simulink model "dc_motor"  (R2022b)
settings: Solver=VariableStepAuto  StartTime=0.0  StopTime=10.0  MaxStep=15e-3  RelTol=1e-3
model workspace (MAT data in the model file):
  J = 7.1e-06
  L_a = 0.0089
  R_a = 5.95
  T_0 = 0.001
  b = 0.001
  k_e = 0.0514
  k_p = 2
  k_t = 0.0514
libraries: simulink x1
settings Model: Creator=Oleg  LastModifiedBy=Oleg
settings DataIOCC: ReturnWorkspaceOutputsName=SDOSimTest_Log
settings DebuggingCC: UnconnectedInputMsg=warning  UnconnectedOutputMsg=warning  UnconnectedLineMsg=warning
settings ModelReferenceCC: EnableRefExpFcnMdlSchedulingChecks=on
settings RTWCC: DLArmComputeVersion=19.05

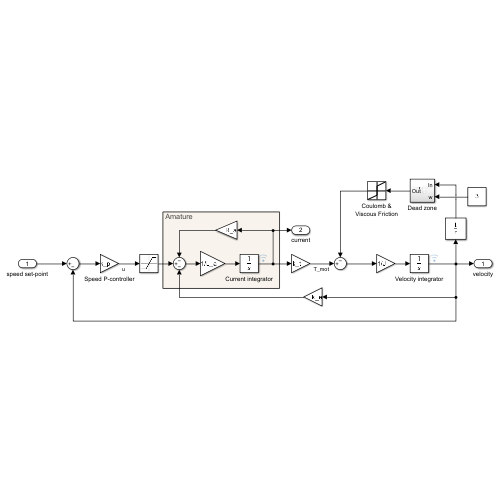
[thumbnail: Simulink's stored preview of the top-level diagram]
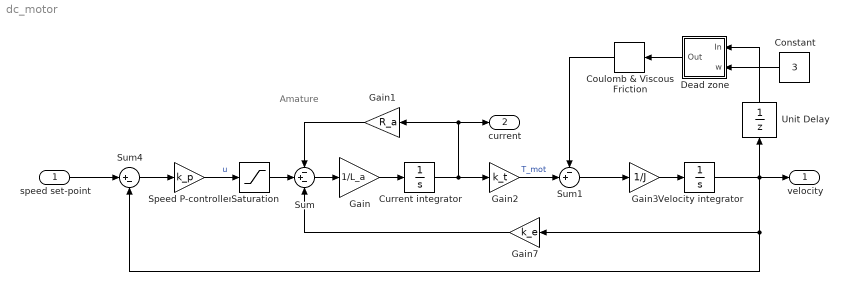
== system dc_motor ==
  note: Amature
  speed set-point : Inport
  Constant : Constant  Value=3
  Coulomb & Viscous Friction : simulink/Discontinuities/Coulomb & Viscous Friction  offset=T_0  gain=b
  Current integrator : Integrator
  Dead zone : Subsystem
  Gain : Gain  Gain=1/L_a
  Gain1 : Gain  Gain=R_a
  Gain2 : Gain  Gain=k_t
  Gain3 : Gain  Gain=1/J
  Gain7 : Gain  Gain=k_e
  Saturation : Saturate  UpperLimit=24  LowerLimit=-24
  Speed P-controller : Gain  Gain=k_p
  Sum : Sum  Inputs=-+-
  Sum1 : Sum  Inputs=-+|
  Sum4 : Sum  Inputs=|+-
  Unit Delay : UnitDelay  SampleTime=-1  HasFrameUpgradeWarning=on
  Velocity integrator : Integrator
  velocity : Outport
  current : Outport  Port=2
  wires:
  Gain/1 -> Current integrator/1
  Sum/1 -> Gain/1
  Gain1/1 -> Sum/1
  Current integrator/1 -> Gain2/1, current/1, Gain1/1
  Gain2/1 -> Sum1/2  "T_mot"
  Sum1/1 -> Gain3/1
  Gain3/1 -> Velocity integrator/1
  Velocity integrator/1 -> Unit Delay/1, velocity/1, Sum4/2, Gain7/1
  Gain7/1 -> Sum/3
  Sum4/1 -> Speed P-controller/1
  Constant/1 -> Dead zone/2(w)
  Unit Delay/1 -> Dead zone/1(In)
  Dead zone/1(Out) -> Coulomb & Viscous Friction/1
  Saturation/1 -> Sum/2
  Speed P-controller/1 -> Saturation/1  "u"
  speed set-point/1 -> Sum4/1
  Coulomb & Viscous Friction/1 -> Sum1/1

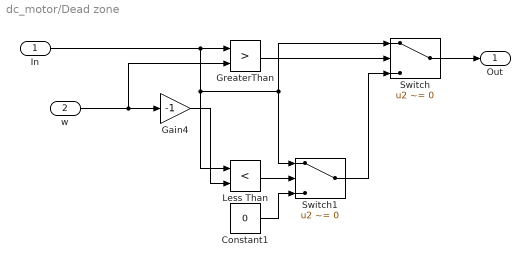
== system dc_motor/Dead zone ==
  In : Inport
  w : Inport  Port=2
  Constant1 : Constant  Value=0
  Gain4 : Gain  Gain=-1
  GreaterThan : RelationalOperator  Operator=>  OutDataTypeStr=boolean  RndMeth=Simplest  InputSameDT=off
  Less Than : RelationalOperator  Operator=<  OutDataTypeStr=boolean  RndMeth=Simplest  InputSameDT=off
  Switch : Switch  Criteria=u2 ~= 0  SaturateOnIntegerOverflow=off  InputSameDT=off
  Switch1 : Switch  Criteria=u2 ~= 0  SaturateOnIntegerOverflow=off  InputSameDT=off
  Out : Outport
  wires:
  w/1 -> Gain4/1, GreaterThan/2
  Switch1/1 -> Switch/3
  Gain4/1 -> Less Than/2
  Switch/1 -> Out/1
  Less Than/1 -> Switch1/2
  GreaterThan/1 -> Switch/2
  In/1 -> Switch/1, Switch1/1, Less Than/1, GreaterThan/1
  Constant1/1 -> Switch1/3
